simulink model "CovidEmBlocos"  (R2021b)
settings: Solver=VariableStepAuto  StartTime=0.0  StopTime=1000  MaxStep=1  RelTol=1e-3
undefined symbols (not defined in the file): beta, I0, r, R0, S0
settings Model: Creator=20.00387-0  LastModifiedBy=20.00387-0

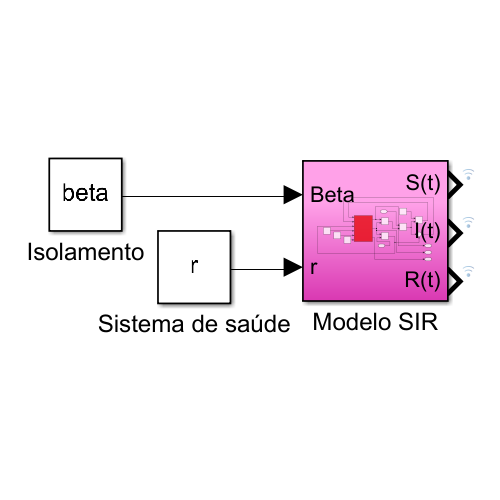
[thumbnail: Simulink's stored preview of the top-level diagram]
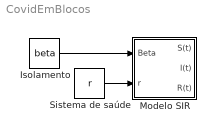
== system CovidEmBlocos ==
  Isolamento : Constant  Value=beta
  Modelo SIR : Subsystem
  Sistema de saúde : Constant  Value=r
  wires:
  Sistema de saúde/1 -> Modelo SIR/2(r)
  Isolamento/1 -> Modelo SIR/1(Beta)

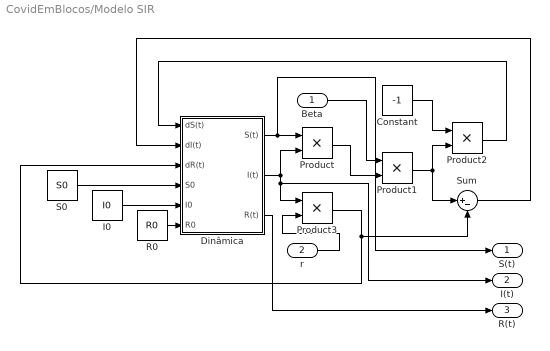
== system CovidEmBlocos/Modelo SIR ==
  Beta : Inport
  r : Inport  Port=2
  Constant : Constant  Value=-1
  Dinâmica : Subsystem
  I0 : Constant  Value=I0
  Product{,1..3} (4 alike) : Product
  R0 : Constant  Value=R0
  S0 : Constant  Value=S0
  Sum : Sum  Inputs=|+-
  S(t) : Outport
  I(t) : Outport  Port=2
  R(t) : Outport  Port=3
  wires:
  Dinâmica/1(S(t)) -> S(t)/1, Product/1
  Product1/1 -> Sum/1, Product2/2
  Product/1 -> Product1/2
  Sum/1 -> Dinâmica/2(dI(t))
  Dinâmica/2(I(t)) -> I(t)/1, Product3/1, Product/2
  R0/1 -> Dinâmica/6(R0)
  Dinâmica/3(R(t)) -> R(t)/1
  Product3/1 -> Sum/2, Dinâmica/3(dR(t))
  Beta/1 -> Product1/1
  r/1 -> Product3/2
  Constant/1 -> Product2/1
  Product2/1 -> Dinâmica/1(dS(t))
  S0/1 -> Dinâmica/4(S0)
  I0/1 -> Dinâmica/5(I0)

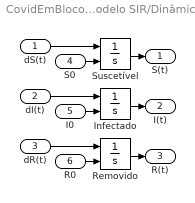
== system CovidEmBlocos/Modelo SIR/Dinâmica ==
  dS(t) : Inport
  dI(t) : Inport  Port=2
  dR(t) : Inport  Port=3
  S0 : Inport  Port=4
  I0 : Inport  Port=5
  R0 : Inport  Port=6
  Infectado : Integrator  InitialConditionSource=external
  Removido : Integrator  InitialConditionSource=external
  Suscetível : Integrator  InitialConditionSource=external
  S(t) : Outport
  I(t) : Outport  Port=2
  R(t) : Outport  Port=3
  wires:
  Infectado/1 -> I(t)/1
  Removido/1 -> R(t)/1
  dS(t)/1 -> Suscetível/1
  Suscetível/1 -> S(t)/1
  dI(t)/1 -> Infectado/1
  S0/1 -> Suscetível/2
  dR(t)/1 -> Removido/1
  I0/1 -> Infectado/2
  R0/1 -> Removido/2
